simulink model "SingleVehicle_01"  (Simulink 8.8)
settings: Solver=VariableStepAuto  StartTime=0.0  StopTime=35  RelTol=1e-3
undefined symbols (not defined in the file or in its folder): ConnectedBus, DiscIntNeverNeededParam, FromPrescan, IdealSensors, psi, x, y
undefined symbols (not defined in the file): vd
libraries: robotlib x3, PreScanUsefulBlocks x1, PreScanSimulinkLibrary x1
settings Model: LogicAnalyzerSignalOrdering=f5e0fbd6-48e8-44a6-8d7f-3c8f77bb7866  Creator=sgopalswamy  LastModifiedBy=sgopalswamy
settings SolverCC: AutoInsertRateTranBlk=on
settings DataIOCC: LimitDataPoints=off  SaveFormat=Dataset  SignalLoggingSaveFormat=Dataset
settings OptimizationCC: LifeSpan=auto
settings DebuggingCC: MultiTaskRateTransMsg=warning  FcnCallInpInsideContextMsg=error  StateNameClashWarn=none  SFUnexpectedBacktrackingDiag=error  SFNoUnconditionalDefaultTransitionDiag=error  SFExecutionAtInitializationDiag=warning
settings HardwareCC: ProdBitPerPointer=64  ProdBitPerSizeT=64  ProdBitPerPtrDiffT=64  ProdLargestAtomicFloat=Float  ProdIntDivRoundTo=Zero  ProdEndianess=LittleEndian  ProdWordSize=64  ProdHWDeviceType=Intel->x86-64 (Windows64)
settings ModelReferenceCC: PropagateSignalLabelsOutOfModel=on
settings GRTTargetCC: TargetLangStandard=C99 (ISO)  GeneratePreprocessorConditionals=Use local settings  CombineOutputUpdateFcns=on  GRTInterface=off
settings ConfigComp: CovMetricSettings=dwe  CovHtmlReporting=off  CovSaveCumulativeToWorkspaceVar=off  CovSaveSingleToWorkspaceVar=off  CovExternalEMLEnable=on

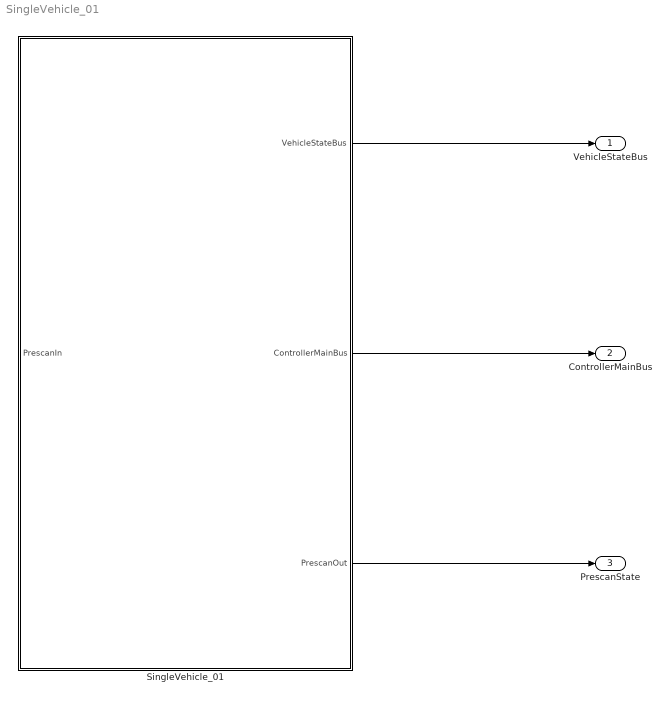
== system SingleVehicle_01 ==
  SingleVehicle_01 : Subsystem  mask{veh_struct=vd}
      mask prompts: veh_struct "Vehicle Parameter Structure"
      mask init:
      | set_param([gcb,'/Monitor/VehicleStateBusStorage'],'VariableName',[get_param(gcb,'MaskValueString'),'_DataVehicleBus']);
      | set_param([gcb,'/Monitor/ControllerMainBusStorage/ArbitratedActuationReqStorage'],'VariableName', ...
      |     [get_param(gcb,'MaskValueString'),'_DataControllerMain_ArbitrationActuationReq']);
      | set_param([gcb,'/Monitor/ControllerMainBusStorage/wpFollowerStorage'],'VariableName', ...
      |     [get_param(gcb,'MaskValueString'),'_DataControllerMain_wpFollower']);
      | set_param([gcb,'/Monitor/ControllerMainBusStorage/finalWayPointStorarge'],'VariableName', ...
      |     [get_param(gcb,'MaskValueString'),'_DataControllerMain_finalWayPoint']);
      | set_param([gcb,'/Monitor/ControllerMainBusStorage/currentWayPointStorage'],'VariableName', ...
      |     [get_param(gcb,'MaskValueString'),'_DataControllerMain_currentWayPoint']);
      | set_param([gcb,'/Monitor/ControllerMainBusStorage/wayPointArrayStorage'],'VariableName', ...
      |     [get_param(gcb,'MaskValueString'),'_DataControllerMain_wayPointArray']);
      | set_param([gcb,'/Monitor/ControllerMainBusStorage/selfAwareessBusStorage'],'VariableName', ...
      |     [get_param(gcb,'MaskValueString'),'_DataControllerMain_selfAwareessBus']);
      | set_param([gcb,'/Monitor/ControllerMainBusStorage/IdealSensorsStorage'],'VariableName', ...
      |     [get_param(gcb,'MaskValueString'),'_DataControllerMain_IdealSensors']);
      | set_param([gcb,'/Monitor/ControllerMainBusStorage/FromPrescanStorage'],'VariableName', ...
      |     [get_param(gcb,'MaskValueString'),'_DataControllerMain_FromPrescan']);
  VehicleStateBus : Outport
  ControllerMainBus : Outport  Port=2
  PrescanState : Outport  Port=3
  wires:
  SingleVehicle_01/1(VehicleStateBus) -> VehicleStateBus/1
  SingleVehicle_01/2(ControllerMainBus) -> ControllerMainBus/1
  SingleVehicle_01/3(PrescanOut) -> PrescanState/1

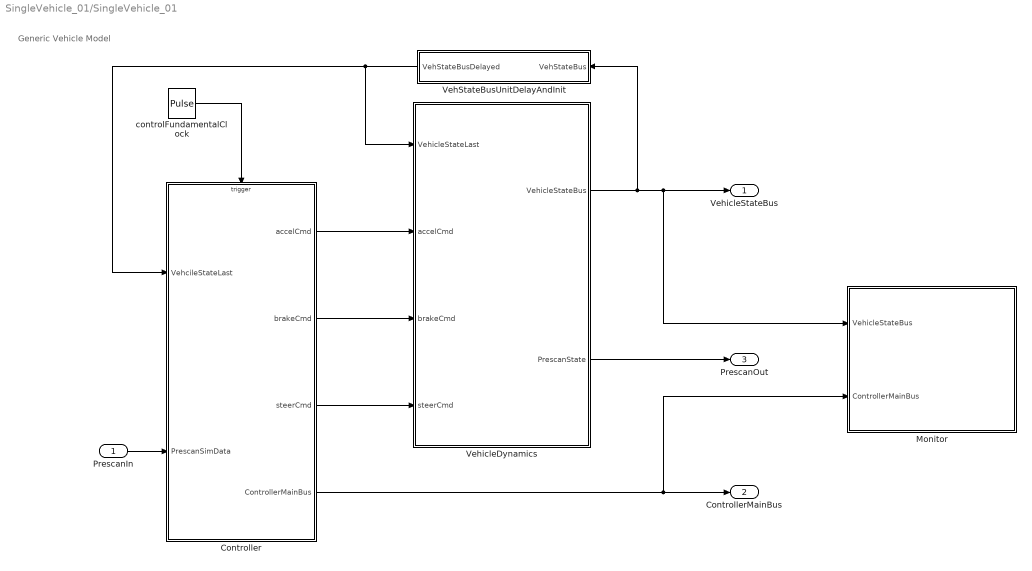
== system SingleVehicle_01/SingleVehicle_01 ==
  note: Generic Vehicle Model
  PrescanIn : Inport
  Controller : Subsystem
  Monitor : Subsystem
  VehStateBusUnitDelayAndInit : Subsystem
  VehicleDynamics : Subsystem
  controlFundamentalClock : DiscretePulseGenerator  PulseType=Time based  Period=veh_struct.CONTROL_OS_SAMPLETIME  PulseWidth=5
  VehicleStateBus : Outport
  ControllerMainBus : Outport  Port=2
  PrescanOut : Outport  Port=3
  wires:
  PrescanIn/1 -> Controller/2(PrescanSimData)
  Controller/1(accelCmd) -> VehicleDynamics/2(accelCmd)
  Controller/2(brakeCmd) -> VehicleDynamics/3(brakeCmd)
  Controller/3(steerCmd) -> VehicleDynamics/4(steerCmd)
  Controller/4(ControllerMainBus) -> Monitor/2(ControllerMainBus), ControllerMainBus/1
  VehicleDynamics/2(PrescanState) -> PrescanOut/1
  VehicleDynamics/1(VehicleStateBus) -> VehStateBusUnitDelayAndInit/1(VehStateBus), VehicleStateBus/1, Monitor/1(VehicleStateBus)
  VehStateBusUnitDelayAndInit/1(VehStateBusDelayed) -> Controller/1(VehcileStateLast), VehicleDynamics/1(VehicleStateLast)
  controlFundamentalClock/1 -> Controller/Trigger

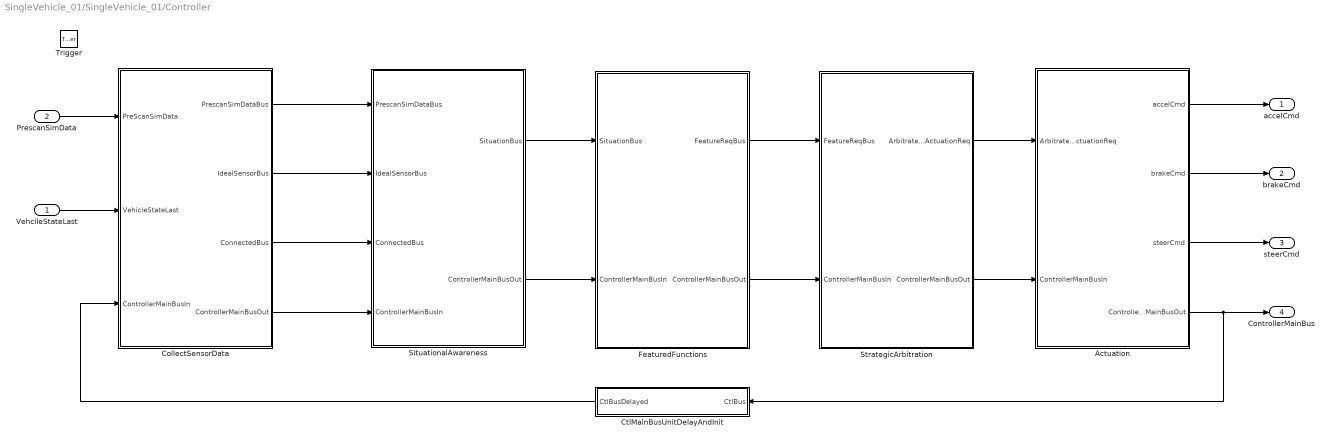
== system SingleVehicle_01/SingleVehicle_01/Controller ==
  VehcileStateLast : Inport
  PrescanSimData : Inport  Port=2
  Trigger : TriggerPort  VariantControl=Variant  PortDimensions=1
  Actuation : Subsystem
  CollectSensorData : Subsystem
  CtlMainBusUnitDelayAndInit : Subsystem
  FeaturedFunctions : Subsystem
  SituationalAwareness : Subsystem
  StrategicArbitration : Subsystem
  accelCmd : Outport
  brakeCmd : Outport  Port=2
  steerCmd : Outport  Port=3
  ControllerMainBus : Outport  Port=4
  wires:
  PrescanSimData/1 -> CollectSensorData/1(PreScanSimData)
  Actuation/1(accelCmd) -> accelCmd/1
  Actuation/2(brakeCmd) -> brakeCmd/1
  Actuation/3(steerCmd) -> steerCmd/1
  StrategicArbitration/1(ArbitratedActuationReq) -> Actuation/1(ArbitratedActuationReq)
  StrategicArbitration/2(ControllerMainBusOut) -> Actuation/2(ControllerMainBusIn)
  FeaturedFunctions/2(ControllerMainBusOut) -> StrategicArbitration/2(ControllerMainBusIn)
  FeaturedFunctions/1(FeatureReqBus) -> StrategicArbitration/1(FeatureReqBus)
  SituationalAwareness/1(SituationBus) -> FeaturedFunctions/1(SituationBus)
  SituationalAwareness/2(ControllerMainBusOut) -> FeaturedFunctions/2(ControllerMainBusIn)
  CollectSensorData/4(ControllerMainBusOut) -> SituationalAwareness/4(ControllerMainBusIn)
  VehcileStateLast/1 -> CollectSensorData/2(VehicleStateLast)
  Actuation/4(ControllerMainBusOut) -> CtlMainBusUnitDelayAndInit/1(CtlBus), ControllerMainBus/1
  CtlMainBusUnitDelayAndInit/1(CtlBusDelayed) -> CollectSensorData/3(ControllerMainBusIn)
  CollectSensorData/1(PrescanSimDataBus) -> SituationalAwareness/1(PrescanSimDataBus)
  CollectSensorData/2(IdealSensorBus) -> SituationalAwareness/2(IdealSensorBus)
  CollectSensorData/3(ConnectedBus) -> SituationalAwareness/3(ConnectedBus)

== system SingleVehicle_01/SingleVehicle_01/Monitor ==
  VehicleStateBus : Inport
  ControllerMainBus : Inport  Port=2
  ControllerMainBusStorage : Subsystem
  VehicleStateBusStorage : ToWorkspace  VariableName=vd_DataVehicleBus  SaveFormat=Timeseries  SampleTime=-1
  wires:
  VehicleStateBus/1 -> VehicleStateBusStorage/1
  ControllerMainBus/1 -> ControllerMainBusStorage/1(ControllerMainBus)

== system SingleVehicle_01/SingleVehicle_01/VehStateBusUnitDelayAndInit ==
  VehStateBus : Inport
  MATLAB Function : MATLAB Function  TreatAsAtomicUnit=on
  Memory : Memory  InheritSampleTime=on
  VehStateBusDelayed : Outport
  wires:
  Memory/1 -> MATLAB Function/1(u)
  VehStateBus/1 -> Memory/1
  MATLAB Function/1(y) -> VehStateBusDelayed/1

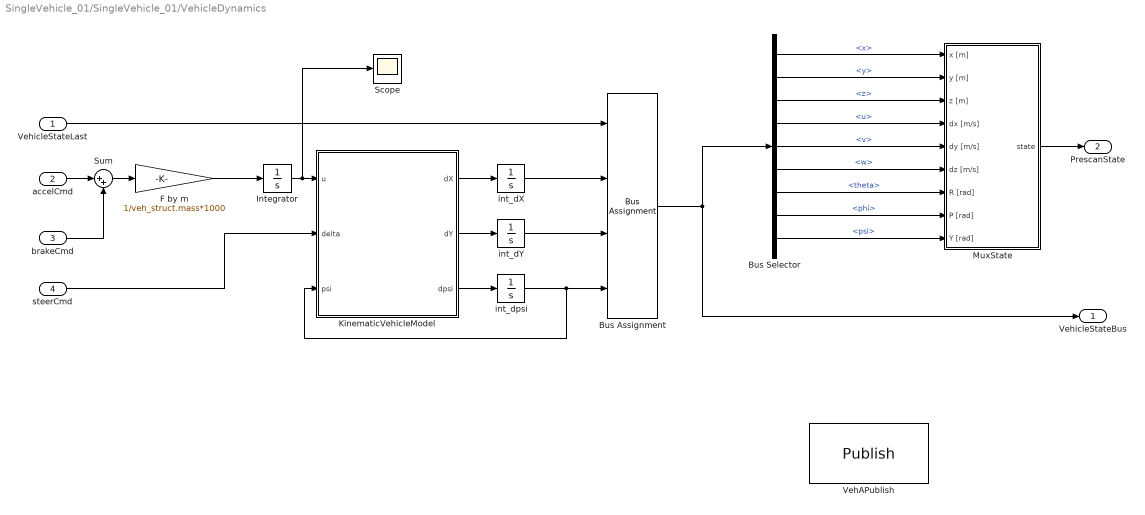
== system SingleVehicle_01/SingleVehicle_01/VehicleDynamics ==
  VehicleStateLast : Inport
  accelCmd : Inport  Port=2
  brakeCmd : Inport  Port=3
  steerCmd : Inport  Port=4
  Bus Assignment : BusAssignment  AssignedSignals=x,y,psi
  Bus Selector : BusSelector  OutputSignals=x,y,z,u,v,w,theta,phi,psi
  F by m : Gain  Gain=1/veh_struct.mass*1000
  Integrator : Integrator  InitialCondition=veh_struct.init.u
  KinematicVehicleModel : MATLAB Function  TreatAsAtomicUnit=on
  MuxState : Subsystem  Tag=MuxState  mask(Empty Dynamics State Block){positioningmode=on, TimeStep=1/20}
      mask prompts: positioningmode "Positioning Mode"; TimeStep "Auto Assigned: Time Step [s]"
      mask help:
      | Build the state of an actor based on user input.
      | The user can either use positioning mode or dynamics mode.
      | - When using positioning mode the position and orientation of the actor are set directly based on the input. Expected input is relative to the initial position and orientation of the actor. It's also possible to specify the velocity of the actor, though this input isn't used, only passed on.
      | - When using dynamics mode the position input is ignored. Expected input is velocity and orientation. The velocity is relative the current orientation of the actor, while orientation is relative to its initial orientation. The position of the actor is calculated based on the velocity and orientation given.
      settings: DeleteFcn=PreScanBlockDeleteFcn;
  Scope : Scope
  Sum : Sum  Inputs=|++
  VehAPublish : robotlib/Publish  SourceLibraryInfo=This block requires Robotics System Toolbox  topicSource=Select from ROS network  topic=/my_topic  messageType=geometry_msgs/Point  messageQueueLength=1
  int_dX : Integrator  InitialCondition=veh_struct.init.X
  int_dY : Integrator  InitialCondition=veh_struct.init.Y
  int_dpsi : Integrator  InitialCondition=veh_struct.init.psi
  VehicleStateBus : Outport
  PrescanState : Outport  Port=2
  wires:
  MuxState/1(state) -> PrescanState/1
  Bus Assignment/1 -> Bus Selector/1, VehicleStateBus/1
  Bus Selector/3 -> MuxState/3(z [m])  "<z>"
  Bus Selector/4 -> MuxState/4(dx [m/s])  "<u>"
  Bus Selector/5 -> MuxState/5(dy [m/s])  "<v>"
  Bus Selector/6 -> MuxState/6(dz [m/s])  "<w>"
  Bus Selector/1 -> MuxState/1(x [m])  "<x>"
  Bus Selector/2 -> MuxState/2(y [m])  "<y>"
  Bus Selector/7 -> MuxState/7(R [rad])  "<theta>"
  Bus Selector/9 -> MuxState/9(Y [rad])  "<psi>"
  Bus Selector/8 -> MuxState/8(P [rad])  "<phi>"
  VehicleStateLast/1 -> Bus Assignment/1
  steerCmd/1 -> KinematicVehicleModel/2(delta)
  accelCmd/1 -> Sum/1
  brakeCmd/1 -> Sum/2
  Sum/1 -> F by m/1
  F by m/1 -> Integrator/1
  Integrator/1 -> Scope/1, KinematicVehicleModel/1(u)
  KinematicVehicleModel/2(dY) -> int_dY/1
  KinematicVehicleModel/1(dX) -> int_dX/1
  KinematicVehicleModel/3(dpsi) -> int_dpsi/1
  int_dX/1 -> Bus Assignment/2
  int_dY/1 -> Bus Assignment/3
  int_dpsi/1 -> Bus Assignment/4, KinematicVehicleModel/3(psi)

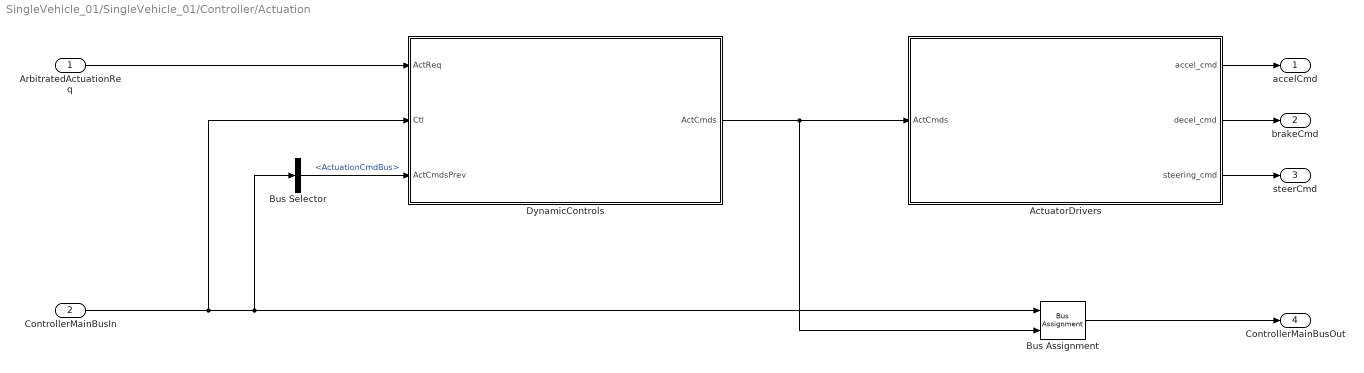
== system SingleVehicle_01/SingleVehicle_01/Controller/Actuation ==
  ArbitratedActuationReq : Inport
  ControllerMainBusIn : Inport  Port=2
  ActuatorDrivers : MATLAB Function  TreatAsAtomicUnit=on
  Bus Assignment : BusAssignment  AssignedSignals=ActuationCmdBus
  Bus Selector : BusSelector  OutputSignals=ActuationCmdBus
  DynamicControls : MATLAB Function  TreatAsAtomicUnit=on
  accelCmd : Outport
  brakeCmd : Outport  Port=2
  steerCmd : Outport  Port=3
  ControllerMainBusOut : Outport  Port=4
  wires:
  ControllerMainBusIn/1 -> DynamicControls/2(Ctl), Bus Assignment/1, Bus Selector/1
  ArbitratedActuationReq/1 -> DynamicControls/1(ActReq)
  Bus Selector/1 -> DynamicControls/3(ActCmdsPrev)  "<ActuationCmdBus>"
  DynamicControls/1(ActCmds) -> ActuatorDrivers/1(ActCmds), Bus Assignment/2
  Bus Assignment/1 -> ControllerMainBusOut/1
  ActuatorDrivers/2(decel_cmd) -> brakeCmd/1
  ActuatorDrivers/1(accel_cmd) -> accelCmd/1
  ActuatorDrivers/3(steering_cmd) -> steerCmd/1

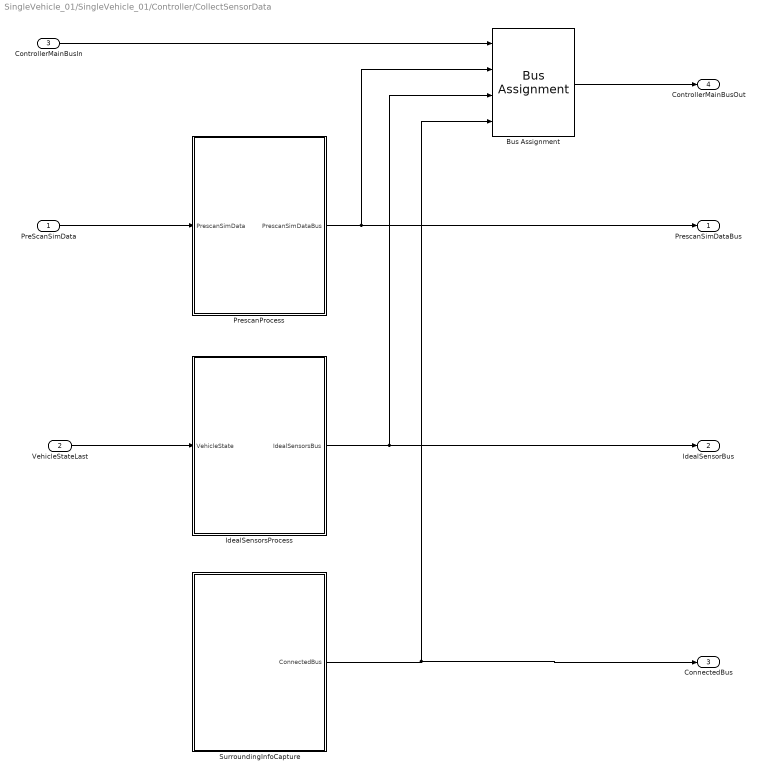
== system SingleVehicle_01/SingleVehicle_01/Controller/CollectSensorData ==
  PreScanSimData : Inport
  VehicleStateLast : Inport  Port=2
  ControllerMainBusIn : Inport  Port=3
  Bus Assignment : BusAssignment  AssignedSignals=FromPrescan,IdealSensors,ConnectedBus
  IdealSensorsProcess : Subsystem
  PrescanProcess : Subsystem
  SurroundingInfoCapture : Subsystem
  PrescanSimDataBus : Outport
  IdealSensorBus : Outport  Port=2
  ConnectedBus : Outport  Port=3
  ControllerMainBusOut : Outport  Port=4
  wires:
  PreScanSimData/1 -> PrescanProcess/1(PrescanSimData)
  PrescanProcess/1(PrescanSimDataBus) -> Bus Assignment/2, PrescanSimDataBus/1
  VehicleStateLast/1 -> IdealSensorsProcess/1(VehicleState)
  IdealSensorsProcess/1(IdealSensorsBus) -> IdealSensorBus/1, Bus Assignment/3
  Bus Assignment/1 -> ControllerMainBusOut/1
  ControllerMainBusIn/1 -> Bus Assignment/1
  SurroundingInfoCapture/1(ConnectedBus) -> ConnectedBus/1, Bus Assignment/4

== system SingleVehicle_01/SingleVehicle_01/Controller/CtlMainBusUnitDelayAndInit ==
  CtlBus : Inport
  MATLAB Function : MATLAB Function  TreatAsAtomicUnit=on
  Memory : Memory  InheritSampleTime=on
  CtlBusDelayed : Outport
  wires:
  Memory/1 -> MATLAB Function/1(u)
  CtlBus/1 -> Memory/1
  MATLAB Function/1(y) -> CtlBusDelayed/1

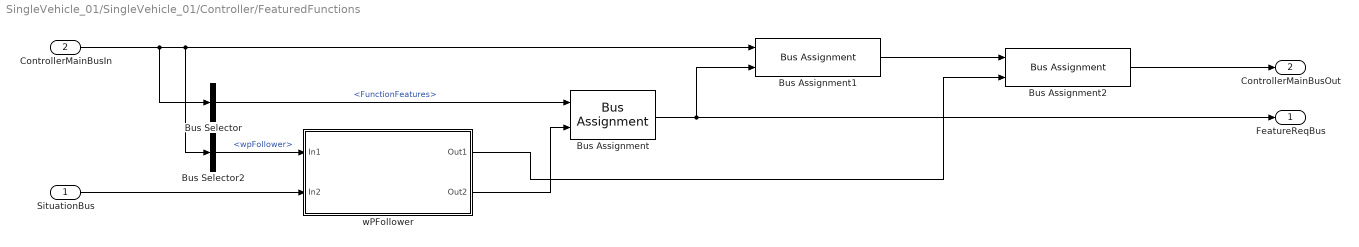
== system SingleVehicle_01/SingleVehicle_01/Controller/FeaturedFunctions ==
  SituationBus : Inport
  ControllerMainBusIn : Inport  Port=2
  Bus Assignment : BusAssignment  AssignedSignals=wpFollower
  Bus Assignment1 : BusAssignment  AssignedSignals=FunctionFeatures
  Bus Assignment2 : BusAssignment  AssignedSignals=situationBus
  Bus Selector : BusSelector  OutputSignals=FunctionFeatures
  Bus Selector2 : BusSelector  OutputSignals=FunctionFeatures.wpFollower
  wPFollower : Subsystem
  FeatureReqBus : Outport
  ControllerMainBusOut : Outport  Port=2
  wires:
  ControllerMainBusIn/1 -> Bus Selector/1, Bus Selector2/1, Bus Assignment1/1
  Bus Selector/1 -> Bus Assignment/1  "<FunctionFeatures>"
  Bus Assignment/1 -> Bus Assignment1/2, FeatureReqBus/1
  Bus Assignment1/1 -> Bus Assignment2/1
  Bus Assignment2/1 -> ControllerMainBusOut/1
  Bus Selector2/1 -> wPFollower/1(In1)  "<wpFollower>"
  SituationBus/1 -> wPFollower/2(In2)
  wPFollower/1(Out1) -> Bus Assignment2/2
  wPFollower/2(Out2) -> Bus Assignment/2

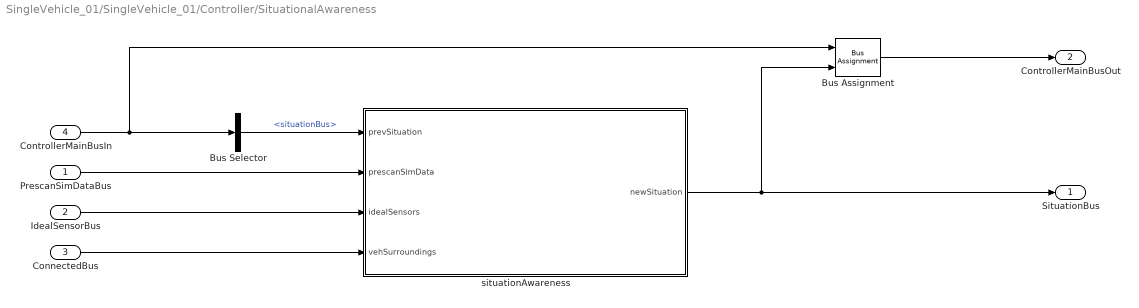
== system SingleVehicle_01/SingleVehicle_01/Controller/SituationalAwareness ==
  PrescanSimDataBus : Inport
  IdealSensorBus : Inport  Port=2
  ConnectedBus : Inport  Port=3
  ControllerMainBusIn : Inport  Port=4
  Bus Assignment : BusAssignment  AssignedSignals=situationBus
  Bus Selector : BusSelector  OutputSignals=situationBus
  situationAwareness : MATLAB Function  TreatAsAtomicUnit=on
  SituationBus : Outport
  ControllerMainBusOut : Outport  Port=2
  wires:
  ControllerMainBusIn/1 -> Bus Assignment/1, Bus Selector/1
  Bus Selector/1 -> situationAwareness/1(prevSituation)  "<situationBus>"
  PrescanSimDataBus/1 -> situationAwareness/2(prescanSimData)
  IdealSensorBus/1 -> situationAwareness/3(idealSensors)
  situationAwareness/1(newSituation) -> Bus Assignment/2, SituationBus/1
  Bus Assignment/1 -> ControllerMainBusOut/1
  ConnectedBus/1 -> situationAwareness/4(vehSurroundings)

== system SingleVehicle_01/SingleVehicle_01/Controller/StrategicArbitration ==
  FeatureReqBus : Inport
  ControllerMainBusIn : Inport  Port=2
  Arbitration : MATLAB Function  TreatAsAtomicUnit=on
  Bus Assignment : BusAssignment  AssignedSignals=ArbitratedActuationReq
  ArbitratedActuationReq : Outport
  ControllerMainBusOut : Outport  Port=2
  wires:
  ControllerMainBusIn/1 -> Bus Assignment/1
  FeatureReqBus/1 -> Arbitration/1(FunctionFeatures)
  Arbitration/1(ArbitratedReq) -> Bus Assignment/2, ArbitratedActuationReq/1
  Bus Assignment/1 -> ControllerMainBusOut/1

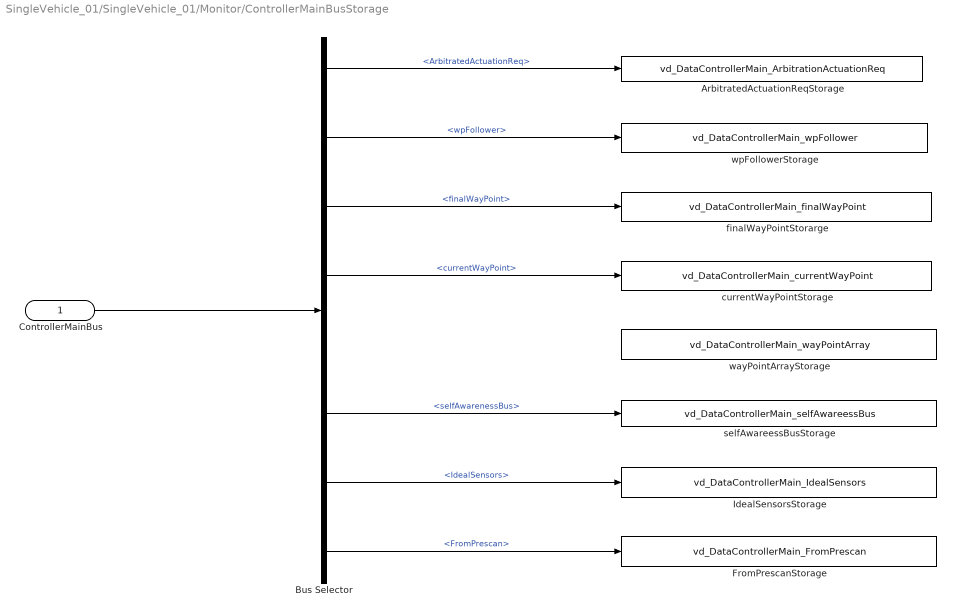
== system SingleVehicle_01/SingleVehicle_01/Monitor/ControllerMainBusStorage ==
  ControllerMainBus : Inport
  ArbitratedActuationReqStorage : ToWorkspace  VariableName=vd_DataControllerMain_ArbitrationActuationReq  SaveFormat=Timeseries  SampleTime=-1
  Bus Selector : BusSelector  OutputSignals=ArbitratedActuationReq,FunctionFeatures.wpFollower,situationBus.wP.finalWayPoint,situationBus.wP.currentWayPoint,situationBus.wP.wayPointArray,situationBus.selfAwarenessBus,IdealSensors,FromPrescan
  FromPrescanStorage : ToWorkspace  VariableName=vd_DataControllerMain_FromPrescan  SaveFormat=Timeseries  SampleTime=-1
  IdealSensorsStorage : ToWorkspace  VariableName=vd_DataControllerMain_IdealSensors  SaveFormat=Timeseries  SampleTime=-1
  currentWayPointStorage : ToWorkspace  VariableName=vd_DataControllerMain_currentWayPoint  SaveFormat=Timeseries  SampleTime=-1
  finalWayPointStorarge : ToWorkspace  VariableName=vd_DataControllerMain_finalWayPoint  SaveFormat=Timeseries  SampleTime=-1
  selfAwareessBusStorage : ToWorkspace  VariableName=vd_DataControllerMain_selfAwareessBus  SaveFormat=Timeseries  SampleTime=-1
  wayPointArrayStorage : ToWorkspace  VariableName=vd_DataControllerMain_wayPointArray  SampleTime=-1
  wpFollowerStorage : ToWorkspace  VariableName=vd_DataControllerMain_wpFollower  SaveFormat=Timeseries  SampleTime=-1
  wires:
  ControllerMainBus/1 -> Bus Selector/1
  Bus Selector/1 -> ArbitratedActuationReqStorage/1  "<ArbitratedActuationReq>"
  Bus Selector/2 -> wpFollowerStorage/1  "<wpFollower>"
  Bus Selector/3 -> finalWayPointStorarge/1  "<finalWayPoint>"
  Bus Selector/8 -> FromPrescanStorage/1  "<FromPrescan>"
  Bus Selector/6 -> selfAwareessBusStorage/1  "<selfAwarenessBus>"
  Bus Selector/4 -> currentWayPointStorage/1  "<currentWayPoint>"
  Bus Selector/7 -> IdealSensorsStorage/1  "<IdealSensors>"

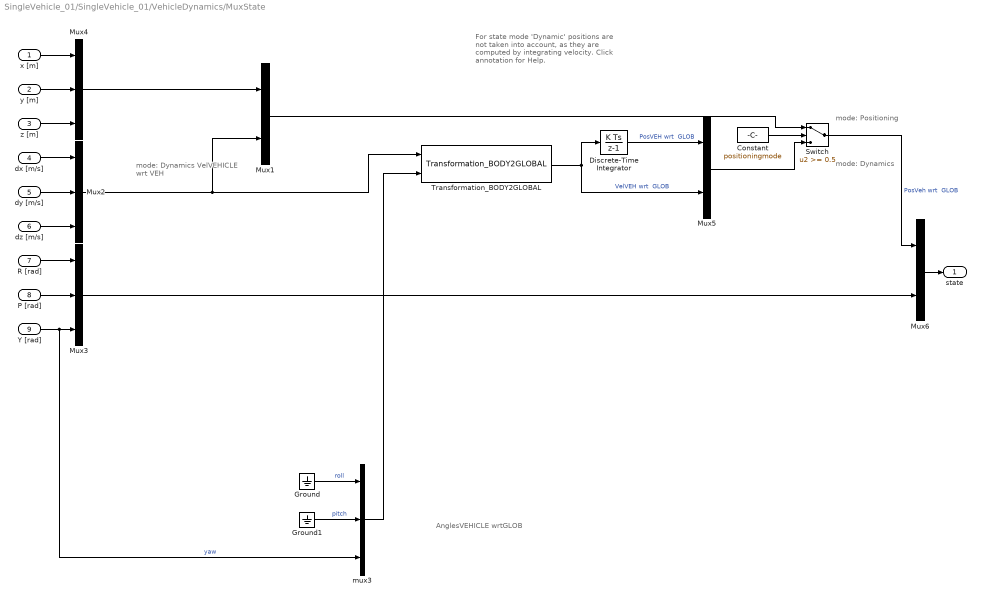
== system SingleVehicle_01/SingleVehicle_01/VehicleDynamics/MuxState ==
  note: mode: Dynamics
  note: mode: Positioning
  note: mode: Dynamics
      | VelVEHICLE
      | wrt VEH
  note: AnglesVEHICLE
      | wrtGLOB
  note: For state mode 'Dynamic' positions
      | are not taken into account, as they
      | are computed by integrating velocity.
      | Click annotation for Help.
  x [m] : Inport  SampleTime=TimeStep
  y [m] : Inport  Port=2  SampleTime=TimeStep
  z [m] : Inport  Port=3  SampleTime=TimeStep
  dx [m/s] : Inport  Port=4  SampleTime=TimeStep
  dy [m/s] : Inport  Port=5  SampleTime=TimeStep
  dz [m/s] : Inport  Port=6  SampleTime=TimeStep
  R [rad] : Inport  Port=7  SampleTime=TimeStep
  P [rad] : Inport  Port=8  SampleTime=TimeStep
  Y [rad] : Inport  Port=9  SampleTime=TimeStep
  Constant : Constant  DisableCoverage=on  Value=positioningmode
  Discrete-Time Integrator : DiscreteIntegrator  SampleTime=TimeStep  ICPrevOutput=DiscIntNeverNeededParam  ICPrevScaledInput=DiscIntNeverNeededParam
  Ground : Ground
  Ground1 : Ground
  Mux1 : Mux  Inputs=[3 3]
  Mux2 : Mux  Inputs=3
  Mux3 : Mux  Inputs=3
  Mux4 : Mux  Inputs=3
  Mux5 : Mux  Inputs=[3 3]
  Mux6 : Mux  Inputs=[6 3]
  Switch : Switch  Threshold=0.5
  Transformation_BODY2GLOBAL : PreScanSimulinkLibrary/Simple_Vehicle_Dynamics/Chassis/MuxDynState/Transformation_BODY2GLOBAL
  mux3 : Mux  Inputs=3
  state : Outport
  wires:
  Constant/1 -> Switch/2
  Mux6/1 -> state/1
  Mux4/1 -> Mux1/1
  Mux5/1 -> Switch/3
  Mux1/1 -> Switch/1
  Switch/1 -> Mux6/1  "PosVeh wrt  GLOB"
  P [rad]/1 -> Mux3/2
  R [rad]/1 -> Mux3/1
  dz [m/s]/1 -> Mux2/3
  dy [m/s]/1 -> Mux2/2
  dx [m/s]/1 -> Mux2/1
  z [m]/1 -> Mux4/3
  y [m]/1 -> Mux4/2
  x [m]/1 -> Mux4/1
  Ground1/1 -> mux3/2  "pitch"
  Y [rad]/1 -> mux3/3, Mux3/3  "yaw"
  Mux3/1 -> Mux6/2
  Transformation_BODY2GLOBAL/1 -> Discrete-Time Integrator/1, Mux5/2  "VelVEH wrt  GLOB"
  mux3/1 -> Transformation_BODY2GLOBAL/2
  Ground/1 -> mux3/1  "roll"
  Mux2/1 -> Mux1/2, Transformation_BODY2GLOBAL/1
  Discrete-Time Integrator/1 -> Mux5/1  "PosVEH wrt  GLOB"

== system SingleVehicle_01/SingleVehicle_01/Controller/CollectSensorData/IdealSensorsProcess ==
  VehicleState : Inport
  Bus Creator : BusCreator  Inputs=12  OutDataTypeStr=Bus: VehState
  Bus Selector : BusSelector  OutputSignals=x,y,z,theta,phi,psi,u,v,w,dtheta,dphi,dpsi
  IdealSensorsBus : Outport
  wires:
  VehicleState/1 -> Bus Selector/1
  Bus Selector/1 -> Bus Creator/1  "<x>"
  Bus Selector/8 -> Bus Creator/8  "<v>"
  Bus Selector/7 -> Bus Creator/7  "<u>"
  Bus Selector/10 -> Bus Creator/10  "<dtheta>"
  Bus Selector/11 -> Bus Creator/11  "<dphi>"
  Bus Selector/6 -> Bus Creator/6  "<psi>"
  Bus Selector/4 -> Bus Creator/4  "<theta>"
  Bus Selector/9 -> Bus Creator/9  "<w>"
  Bus Selector/2 -> Bus Creator/2  "<y>"
  Bus Selector/5 -> Bus Creator/5  "<phi>"
  Bus Selector/12 -> Bus Creator/12  "<dpsi>"
  Bus Selector/3 -> Bus Creator/3  "<z>"
  Bus Creator/1 -> IdealSensorsBus/1

== system SingleVehicle_01/SingleVehicle_01/Controller/CollectSensorData/PrescanProcess ==
  PrescanSimData : Inport
  Bus Creator : BusCreator  Inputs=12  OutDataTypeStr=Bus: PrescanSimData
      settings: InheritFromInputs=off
  SELF_Demux : Subsystem  Tag=DemuxSELF  mask(PreScan Demux Block:){}
      settings: DeleteFcn=PreScanBlockDeleteFcn;
      mask Display:
      | port_label('output',1,'x [m]')
      | port_label('output',2,'y [m]')
      | port_label('output',3,'z [m]','texmode','on')
      | port_label('output',4,'Rotx [deg]','texmode','on')
      | port_label('output',5,'Roty [deg]','texmode','on')
      | port_label('output',6,'Rotz [deg]','texmode','on')
      | port_label('output',7,'GPS lat [deg]','texmode','on')
      | port_label('output',8,'GPS long [deg]','texmode','on')
      | port_label('output',9,'GPS alt [m]','texmode','on')
      | port_label('output',10,'Velocity [m/s]')
      | port_label('output',11,'Heading [deg]')
      | port_label('output',12,'Yaw rate [deg/s]')
  PrescanSimDataBus : Outport
  wires:
  SELF_Demux/1(x [m]) -> Bus Creator/1  "x"
  PrescanSimData/1 -> SELF_Demux/1(SELF)
  Bus Creator/1 -> PrescanSimDataBus/1
  SELF_Demux/2(y [m]) -> Bus Creator/2  "y"
  SELF_Demux/3(z [m]) -> Bus Creator/3  "z"
  SELF_Demux/4(rotx [deg]) -> Bus Creator/4  "Rotx"
  SELF_Demux/5(roty [deg]) -> Bus Creator/5  "Roty"
  SELF_Demux/9(GPS alt [m]) -> Bus Creator/9  "GPS_alt"
  SELF_Demux/8(GPS long [deg]) -> Bus Creator/8  "GPS_long"
  SELF_Demux/10(velocity [m/s]) -> Bus Creator/10  "u"
  SELF_Demux/6(rotz [deg]) -> Bus Creator/6  "Rotz"
  SELF_Demux/7(GPS lat [deg]) -> Bus Creator/7  "GPS_lat"
  SELF_Demux/11(heading [deg]) -> Bus Creator/11  "heading"
  SELF_Demux/12(yaw rate [deg/s]) -> Bus Creator/12  "Yaw_rate"

== system SingleVehicle_01/SingleVehicle_01/Controller/CollectSensorData/SurroundingInfoCapture ==
  Bus Creator : BusCreator  Inputs=2  OutDataTypeStr=Bus: ConnectedBus
  Bus Creator1 : BusCreator  Inputs=3  OutDataTypeStr=Bus: ObjectBus
  Bus Selector1 : BusSelector  OutputSignals=X,Y,Z
  NumberObject : Constant  Value=2
  Terminator : Terminator
  VehicleB_FromSim_Object2 : robotlib/Subscribe  SourceLibraryInfo=This block requires Robotics System Toolbox  topicSource=Select from ROS network  topic=/my_topic  messageType=geometry_msgs/Point  sampleTime=-1  messageQueueLength=1
  VehicleC_RCVehicle_Object1 : robotlib/Subscribe  SourceLibraryInfo=This block requires Robotics System Toolbox  topicSource=Select from ROS network  topic=/my_topic  messageType=geometry_msgs/Point  sampleTime=-1  messageQueueLength=1
  ConnectedBus : Outport
  wires:
  Bus Creator/1 -> ConnectedBus/1
  VehicleC_RCVehicle_Object1/2 -> Bus Selector1/1
  Bus Selector1/1 -> Bus Creator1/1  "<X>"
  Bus Selector1/2 -> Bus Creator1/2  "<Y>"
  Bus Selector1/3 -> Bus Creator1/3  "<Z>"
  NumberObject/1 -> Bus Creator/2  "NumberObjects"
  VehicleC_RCVehicle_Object1/1 -> Terminator/1
  Bus Creator1/1 -> Bus Creator/1  "ObjectBus"

== system SingleVehicle_01/SingleVehicle_01/Controller/FeaturedFunctions/wPFollower ==
  In1 : Inport
  In2 : Inport  Port=2
  calcDesdCmds : MATLAB Function  TreatAsAtomicUnit=on
  defineWayPointsNewWay : MATLAB Function  TreatAsAtomicUnit=on
  defineWayPointsOldWay : MATLAB Function  TreatAsAtomicUnit=on
  Out1 : Outport
  Out2 : Outport  Port=2
  wires:
  In2/1 -> defineWayPointsOldWay/2(prevSituation)
  In1/1 -> defineWayPointsOldWay/1(prevWpAction)
  defineWayPointsOldWay/1(wpAction) -> Out2/1
  defineWayPointsOldWay/2(newSituation) -> Out1/1

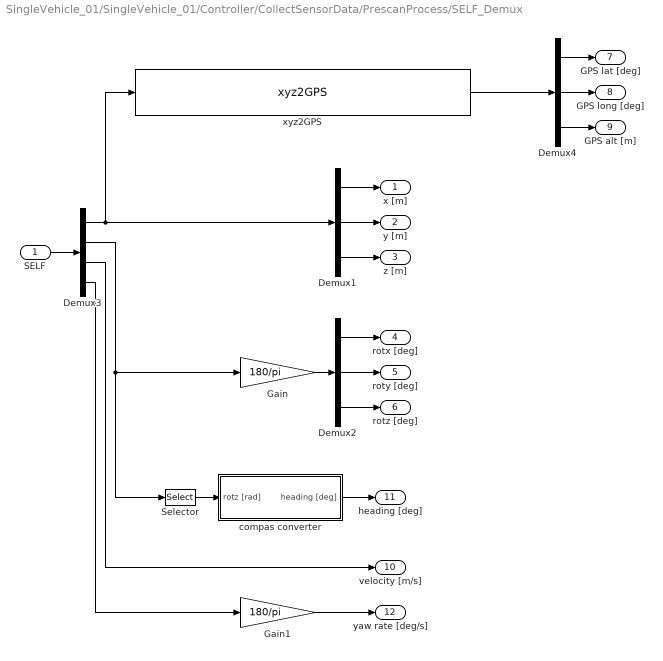
== system SingleVehicle_01/SingleVehicle_01/Controller/CollectSensorData/PrescanProcess/SELF_Demux ==
  SELF : Inport
  Demux1 : Demux  Outputs=3
  Demux2 : Demux  Outputs=3
  Demux3 : Demux  Outputs=[3 3 1 1]
  Demux4 : Demux  Outputs=3
  Gain : Gain  Gain=180/pi
  Gain1 : Gain  Gain=180/pi
  Selector : Selector  InputPortWidth=3  IndexOptions=Index vector (dialog)  Indices=[3]  OutputSizes=1
  compas converter : Subsystem
  xyz2GPS : PreScanUsefulBlocks/xyz2GPS  CoordinateCount=1  GPS_base=[0.000000 0.000000 0.000]
  x [m] : Outport
  y [m] : Outport  Port=2
  z [m] : Outport  Port=3
  rotx [deg] : Outport  Port=4
  roty [deg] : Outport  Port=5
  rotz [deg] : Outport  Port=6
  GPS lat [deg] : Outport  Port=7
  GPS long [deg] : Outport  Port=8
  GPS alt [m] : Outport  Port=9
  velocity [m/s] : Outport  Port=10
  heading [deg] : Outport  Port=11
  yaw rate [deg/s] : Outport  Port=12
  wires:
  Demux3/4 -> Gain1/1
  Gain1/1 -> yaw rate [deg/s]/1
  Demux3/3 -> velocity [m/s]/1
  compas converter/1(heading [deg]) -> heading [deg]/1
  xyz2GPS/1 -> Demux4/1
  Demux4/3 -> GPS alt [m]/1
  Demux4/2 -> GPS long [deg]/1
  Demux4/1 -> GPS lat [deg]/1
  Demux3/2 -> Gain/1, Selector/1
  Demux3/1 -> xyz2GPS/1, Demux1/1
  SELF/1 -> Demux3/1
  Demux2/3 -> rotz [deg]/1
  Demux2/2 -> roty [deg]/1
  Demux2/1 -> rotx [deg]/1
  Demux1/3 -> z [m]/1
  Demux1/2 -> y [m]/1
  Demux1/1 -> x [m]/1
  Gain/1 -> Demux2/1
  Selector/1 -> compas converter/1(rotz [rad])

== system SingleVehicle_01/SingleVehicle_01/Controller/CollectSensorData/PrescanProcess/SELF_Demux/compas converter ==
  rotz [rad] : Inport
  cart2compas : Subsystem
  rad2deg : Gain  Gain=180/pi
  heading [deg] : Outport
  wires:
  cart2compas/1(heading [deg]) -> heading [deg]/1
  rotz [rad]/1 -> rad2deg/1
  rad2deg/1 -> cart2compas/1(Angle [deg])

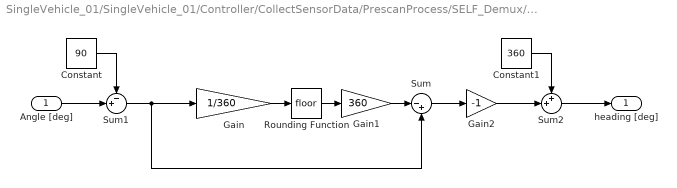
== system SingleVehicle_01/SingleVehicle_01/Controller/CollectSensorData/PrescanProcess/SELF_Demux/compas converter/cart2compas ==
  Angle [deg] : Inport
  Constant : Constant  Value=90
  Constant1 : Constant  Value=360
  Gain : Gain  Gain=1/360
  Gain1 : Gain  Gain=360
  Gain2 : Gain  Gain=-1
  Rounding Function : Rounding
  Sum : Sum  Inputs=|-+
  Sum1 : Sum  Inputs=-+|
  Sum2 : Sum  Inputs=++|
  heading [deg] : Outport
  wires:
  Sum2/1 -> heading [deg]/1
  Constant1/1 -> Sum2/1
  Gain2/1 -> Sum2/2
  Constant/1 -> Sum1/1
  Sum1/1 -> Sum/2, Gain/1
  Sum/1 -> Gain2/1
  Angle [deg]/1 -> Sum1/2
  Gain1/1 -> Sum/1
  Rounding Function/1 -> Gain1/1
  Gain/1 -> Rounding Function/1

== matlab function SingleVehicle_01/Controller/CtlMainBusUnitDelayAndInit/MATLAB Function ==
  data: u input double; y output Bus: ControllerMainBus; veh_struct parameter double
function y = DelayAndInitCtlBus(u, veh_struct)
coder.extrinsic('exist')
persistent a

y0 = struct;

y0.ActuationCmdBus = struct;
y0.ActuationCmdBus.steering_cmd = 0;
y0.ActuationCmdBus.decel_cmd = 0;
y0.ActuationCmdBus.accel_cmd = 0;

y0.ArbitratedActuationReq = struct;
y0.ArbitratedActuationReq.v_des = 0;
y0.ArbitratedActuationReq.a_des = 0;
y0.ArbitratedActuationReq.psi_des = 0;
y0.ArbitratedActuationReq.dpsi_des = 0;


y0.FunctionFeatures = struct;
y0.FunctionFeatures.wpFollower = struct;
y0.FunctionFeatures.wpFollower.v_des = 0;
y0.FunctionFeatures.wpFollower.a_des = 0;
y0.FunctionFeatures.wpFollower.psi_des = 0;
y0.FunctionFeatures.wpFollower.dpsi_des = 0;


y0.situationBus = struct;
y0.situationBus.wP = struct;

y0.situationBus.wP.finalWayPoint = struct;
y0.situationBus.wP.finalWayPoint.x = 0;
y0.situationBus.wP.finalWayPoint.y = 0;
y0.situationBus.wP.finalWayPoint.z = 0;
y0.situationBus.wP.finalWayPoint.treach = 0;

y0.situationBus.wP.currentWayPoint = struct;
y0.situationBus.wP.currentWayPoint.x = 0;
y0.situationBus.wP.currentWayPoint.y = 0;
y0.situationBus.wP.currentWayPoint.z = 0;
y0.situationBus.wP.currentWayPoint.treach = 0;

y0.situationBus.wP.finalWayPointIndex = uint16(1);
y0.situationBus.wP.currentWayPointIndex = uint16(10);

%y0.situationBus.wP.wayPointArray = struct;
wPArray = struct;
wPArray.x = 0;
wPArray.y = 0;
wPArray.z = 0;
wPArray.treach = 0;
y0.situationBus.wP.wayPointArray = repmat(wPArray,100,1);


y0.situationBus.selfAwarenessBus = struct;
y0.situationBus.selfAwarenessBus.x = 0;
y0.situationBus.selfAwarenessBus.y = 0;
y0.situationBus.selfAwarenessBus.z = 0;
y0.situationBus.selfAwarenessBus.theta = 0;
y0.situationBus.selfAwarenessBus.phi = 0;
y0.situationBus.selfAwarenessBus.psi = 0;
y0.situationBus.selfAwarenessBus.u = 0;
y0.situationBus.selfAwarenessBus.v = 0;
y0.situationBus.selfAwarenessBus.w = 0;
y0.situationBus.selfAwarenessBus.dtheta = 0;
y0.situationBus.selfAwarenessBus.dphi = 0;
y0.situationBus.selfAwarenessBus.dpsi = 0;
y0.IdealSensors = struct;
y0.IdealSensors.x = 0;
y0.IdealSensors.y = 0;
y0.IdealSensors.z = 0;
y0.IdealSensors.theta = 0;
y0.IdealSensors.phi = 0;
y0.IdealSensors.psi = 0;
y0.IdealSensors.u = 0;
y0.IdealSensors.v = 0;
y0.IdealSensors.w = 0;
y0.IdealSensors.dtheta = 0;
y0.IdealSensors.dphi = 0;
y0.IdealSensors.dpsi = 0;
y0.FromPrescan = struct;
y0.FromPrescan.x = 0;
y0.FromPrescan.y = 0;
y0.FromPrescan.z = 0;
y0.FromPrescan.Rotx = 0;
y0.FromPrescan.Roty = 0;
y0.FromPrescan.Rotz = 0;
y0.FromPrescan.GPS_lat = 0;
y0.FromPrescan.GPS_long = 0;
y0.FromPrescan.u = 0;
y0.FromPrescan.GPS_alt = 0;
y0.FromPrescan.heading = 0;
y0.FromPrescan.Yaw_rate = 0;

y0.ConnectedBus = struct;
y0.ConnectedBus.ObjectBus = struct;
y0.ConnectedBus.ObjectBus.x = 0;
y0.ConnectedBus.ObjectBus.y = 0;
y0.ConnectedBus.ObjectBus.z = 0;
y0.ConnectedBus.NumberObjects = 0;



if isempty(a)
    a = 1;
    y = y0;
    y.situationBus.wP.wayPointArray = veh_struct.initialWayPointsArray;
    y.situationBus.wP.currentWayPointIndex = veh_struct.initialCurrentWayPointIndex;
    y.situationBus.wP.finalWayPointIndex = veh_struct.initialFinalWayPointIndex;

else
    y = u;
end

== matlab function SingleVehicle_01/VehStateBusUnitDelayAndInit/MATLAB Function ==
  data: u input double; y output Bus: VehState
function y = DelayAndInitVehState(u)
persistent a
y0 = struct;
y0.x = 1;
y0.y = 2;
y0.z = 0;
y0.theta = 0;
y0.phi = 0;
y0.psi = 0;
y0.u = 0;
y0.v = 0;
y0.w = 0;
y0.dtheta = 0;
y0.dphi = 0;
y0.dpsi = 0;

%y0 = VehState_MATLABStruct;
if isempty(a)
    a = 1;
    y = y0;
else
    y = u;
end

== matlab function SingleVehicle_01/Controller/SituationalAwareness/situationAwareness ==
  data: prevSituation input Bus: situationBus; newSituation output Bus: situationBus; prescanSimData input Bus: PrescanSimData; idealSensors input Bus: VehState; veh_struct parameter double; vehSurroundings input double
function newSituation = calcSituationAwareness(prevSituation,prescanSimData,idealSensors, veh_struct, vehSurroundings)

newSituation = prevSituation;


newSituation.selfAwarenessBus.x = idealSensors.x;
newSituation.selfAwarenessBus.y = idealSensors.y;
newSituation.selfAwarenessBus.z = idealSensors.z;
newSituation.selfAwarenessBus.theta = idealSensors.theta;
newSituation.selfAwarenessBus.phi = idealSensors.phi;
newSituation.selfAwarenessBus.psi = idealSensors.psi;
newSituation.selfAwarenessBus.u = idealSensors.u;
newSituation.selfAwarenessBus.v = idealSensors.v;
newSituation.selfAwarenessBus.w = idealSensors.w;
newSituation.selfAwarenessBus.dtheta = idealSensors.dtheta;
newSituation.selfAwarenessBus.dphi = idealSensors.dphi;
newSituation.selfAwarenessBus.dpsi = idealSensors.dpsi;

for i = 1: ContorllerBus.ConnectedBus.NumberObjects
    newSituation.contextualAwareness.ObjectBus(1).x = ControllerBus.ConnectedBus.ObjectBus(1).x;
    newSituation.contextualAwareness.ObjectBus(1).x = ControllerBus.ConnectedBus.ObjectBus(1).y;
    newSituation.contextualAwareness.ObjectBus(1).x = ControllerBus.ConnectedBus.ObjectBus(1).z;
end


end

== matlab function SingleVehicle_01/Controller/FeaturedFunctions/wPFollower/defineWayPointsOldWay ==
  data: prevWpAction input Bus: wpFollower; prevSituation input Bus: situationBus; wpAction output Bus: wpFollower; veh_struct parameter double; newSituation output Bus: situationBus
function [wpAction, newSituation] = wpFollower(prevWpAction, prevSituation, veh_struct)


%waypoint Definition
currentIndex = prevSituation.wP.currentWayPointIndex;
if currentIndex < 1
    currentIndex = uint16(1);
end
finalIndex = prevSituation.wP.finalWayPointIndex;

xd = prevSituation.wP.wayPointArray(currentIndex).x;
yd = prevSituation.wP.wayPointArray(currentIndex).y;
xa = prevSituation.selfAwarenessBus.x;
ya = prevSituation.selfAwarenessBus.y;
howClose = norm([xd-xa, yd-ya]);

if howClose < veh_struct.wpControl.wayPointThreshold
    if (currentIndex == finalIndex)
        currentIndex = uint16(1);
    else
        currentIndex = uint16(currentIndex + 1);
    end
end

newSituation = prevSituation;
newSituation.wP.currentWayPointIndex = uint16(currentIndex);
newSituation.wP.currentWayPoint.x = newSituation.wP.wayPointArray(currentIndex).x;
newSituation.wP.currentWayPoint.y = newSituation.wP.wayPointArray(currentIndex).y;
newSituation.wP.currentWayPoint.z = newSituation.wP.wayPointArray(currentIndex).z;
newSituation.wP.currentWayPoint.treach = newSituation.wP.wayPointArray(currentIndex).treach;


%New Way POint Definition

newSituation = prevSituation;
newSituation.wP.currentWayPointIndex = uint16(currentIndex);
newSituation.wP.currentWayPoint.x = ControllerBus.ConnectedBus.ObjectBus.x;
newSituation.wP.currentWayPoint.y = ControllerBus.ConnectedBus.ObjectBus.y;
newSituation.wP.currentWayPoint.z = ControllerBus.ConnectedBus.ObjectBus.z;
newSituation.wP.currentWayPoint.treach = 0;


%wayPoint Following Algorithm

v_des_raw = min(veh_struct.wpControl.v_des_max, howClose / veh_struct.wpControl.howClose_saturate * veh_struct.wpControl.v_des_max);
psi_des_raw = atan2((yd-ya),(xd-xa));

% if psi_des_raw < 0
%     
%     dbg = 1;
%     
% end
    

v_des_old = prevWpAction.v_des;
psi_des_old = prevWpAction.psi_des;

a_des = veh_struct.wpControl.v_des_filter.lambda * (v_des_raw - v_des_old);
v_des = v_des_old + veh_struct.CONTROL_OS_SAMPLETIME * a_des;

dpsi_des = veh_struct.wpControl.psi_des_filter.lambda * (psi_des_raw - psi_des_old);
psi_des = psi_des_old + veh_struct.CONTROL_OS_SAMPLETIME * dpsi_des;
% psi_des = mod(psi_des, 2 * pi);


wpAction.v_des = v_des;
wpAction.a_des = a_des;
wpAction.psi_des = psi_des;
wpAction.dpsi_des = dpsi_des;

end

== matlab function SingleVehicle_01/Controller/StrategicArbitration/Arbitration ==
  data: FunctionFeatures input Bus: FunctionFeatures; ArbitratedReq output Bus: ArbitratedActuationReq
function ArbitratedReq = Arbitrate(FunctionFeatures)

ArbitratedReq.v_des = FunctionFeatures.wpFollower.v_des;
ArbitratedReq.a_des = FunctionFeatures.wpFollower.a_des;
ArbitratedReq.psi_des = FunctionFeatures.wpFollower.psi_des;
ArbitratedReq.dpsi_des = FunctionFeatures.wpFollower.dpsi_des;

end

== matlab function SingleVehicle_01/Controller/Actuation/DynamicControls ==
  data: ActReq input Bus: ArbitratedActuationReq; Ctl input Bus: ControllerMainBus; ActCmds output Bus: ActuationCmdBus; ActCmdsPrev input Bus: ActuationCmdBus
function ActCmds  = fcn(ActReq, Ctl, ActCmdsPrev)

v_des = ActReq.v_des;
a_des = ActReq.a_des;
psi_des = ActReq.psi_des;
dpsi_des = ActReq.dpsi_des;

% ActCmds = ActCmdsPrev;
% ActCmds.accel_cmd = 0;
% ActCmds.decel_cmd = 0;
% ActCmds.steering_cmd = 0.1;

ActCmds = ActCmdsPrev;

if a_des >= 0
    ActCmds.accel_cmd = ActReq.a_des;
    ActCmds.decel_cmd = 0;
else
    ActCmds.accel_cmd = 0;
    ActCmds.decel_cmd = ActReq.a_des;
end

psi_des = unwrap(psi_des);
Ctl.IdealSensors.psi = unwrap(Ctl.IdealSensors.psi);

ActCmds.steering_cmd = 3.5*(psi_des - Ctl.IdealSensors.psi);

== matlab function SingleVehicle_01/VehicleDynamics/KinematicVehicleModel ==
  data: u input double; delta input double; dX output double; psi input double; dY output double; dpsi output double; veh_struct parameter double
function [dX,dY,dpsi] = fcn(u,delta, psi, veh_struct)

lf = veh_struct.lf;
lr = veh_struct.lr;

% psi = unwrap(psi);
% delta = unwrap(delta);

beta = atan( lr /(lf + lr) * tan(delta));

% beta = unwrap(beta);

dX = u * cos(psi + beta);
dY = u * sin(psi + beta);
dpsi = u / lr * sin(beta);

== matlab function SingleVehicle_01/Controller/Actuation/ActuatorDrivers ==
  data: ActCmds input Bus: ActuationCmdBus; accel_cmd output double; decel_cmd output double; steering_cmd output double
function [accel_cmd, decel_cmd, steering_cmd]  = fcn(ActCmds)

accel_cmd = ActCmds.accel_cmd;
decel_cmd = ActCmds.decel_cmd;
steering_cmd = ActCmds.steering_cmd;

end

== matlab function SingleVehicle_01/Controller/FeaturedFunctions/wPFollower/calcDesdCmds ==
  data: prevWpAction input Bus: wpFollower; prevSituation input Bus: situationBus; wpAction output Bus: wpFollower; veh_struct parameter double; newSituation output Bus: situationBus
function [wpAction, newSituation] = wpFollower(prevWpAction, prevSituation, veh_struct)


%waypoint Definition
currentIndex = prevSituation.wP.currentWayPointIndex;
if currentIndex < 1
    currentIndex = uint16(1);
end
finalIndex = prevSituation.wP.finalWayPointIndex;

xd = prevSituation.wP.wayPointArray(currentIndex).x;
yd = prevSituation.wP.wayPointArray(currentIndex).y;
xa = prevSituation.selfAwarenessBus.x;
ya = prevSituation.selfAwarenessBus.y;
howClose = norm([xd-xa, yd-ya]);

if howClose < veh_struct.wpControl.wayPointThreshold
    if (currentIndex == finalIndex)
        currentIndex = uint16(1);
    else
        currentIndex = uint16(currentIndex + 1);
    end
end

newSituation = prevSituation;
newSituation.wP.currentWayPointIndex = uint16(currentIndex);
newSituation.wP.currentWayPoint.x = newSituation.wP.wayPointArray(currentIndex).x;
newSituation.wP.currentWayPoint.y = newSituation.wP.wayPointArray(currentIndex).y;
newSituation.wP.currentWayPoint.z = newSituation.wP.wayPointArray(currentIndex).z;
newSituation.wP.currentWayPoint.treach = newSituation.wP.wayPointArray(currentIndex).treach;


%New Way POint Definition

newSituation = prevSituation;
newSituation.wP.currentWayPointIndex = uint16(currentIndex);
newSituation.wP.currentWayPoint.x = ControllerBus.ConnectedBus.ObjectBus.x;
newSituation.wP.currentWayPoint.y = ControllerBus.ConnectedBus.ObjectBus.y;
newSituation.wP.currentWayPoint.z = ControllerBus.ConnectedBus.ObjectBus.z;
newSituation.wP.currentWayPoint.treach = 0;


%wayPoint Following Algorithm

v_des_raw = min(veh_struct.wpControl.v_des_max, howClose / veh_struct.wpControl.howClose_saturate * veh_struct.wpControl.v_des_max);
psi_des_raw = atan2((yd-ya),(xd-xa));

% if psi_des_raw < 0
%     
%     dbg = 1;
%     
% end
    

v_des_old = prevWpAction.v_des;
psi_des_old = prevWpAction.psi_des;

a_des = veh_struct.wpControl.v_des_filter.lambda * (v_des_raw - v_des_old);
v_des = v_des_old + veh_struct.CONTROL_OS_SAMPLETIME * a_des;

dpsi_des = veh_struct.wpControl.psi_des_filter.lambda * (psi_des_raw - psi_des_old);
psi_des = psi_des_old + veh_struct.CONTROL_OS_SAMPLETIME * dpsi_des;
% psi_des = mod(psi_des, 2 * pi);


wpAction.v_des = v_des;
wpAction.a_des = a_des;
wpAction.psi_des = psi_des;
wpAction.dpsi_des = dpsi_des;

end

== matlab function SingleVehicle_01/Controller/FeaturedFunctions/wPFollower/defineWayPointsNewWay ==
  data: prevWpAction input Bus: wpFollower; prevSituation input Bus: situationBus; wpAction output Bus: wpFollower; veh_struct parameter double; newSituation output Bus: situationBus
function [wpAction, newSituation] = wpFollower(prevWpAction, prevSituation, veh_struct)


%waypoint Definition
currentIndex = prevSituation.wP.currentWayPointIndex;
if currentIndex < 1
    currentIndex = uint16(1);
end
finalIndex = prevSituation.wP.finalWayPointIndex;

xd = prevSituation.wP.wayPointArray(currentIndex).x;
yd = prevSituation.wP.wayPointArray(currentIndex).y;
xa = prevSituation.selfAwarenessBus.x;
ya = prevSituation.selfAwarenessBus.y;
howClose = norm([xd-xa, yd-ya]);

if howClose < veh_struct.wpControl.wayPointThreshold
    if (currentIndex == finalIndex)
        currentIndex = uint16(1);
    else
        currentIndex = uint16(currentIndex + 1);
    end
end

newSituation = prevSituation;
newSituation.wP.currentWayPointIndex = uint16(currentIndex);
newSituation.wP.currentWayPoint.x = newSituation.wP.wayPointArray(currentIndex).x;
newSituation.wP.currentWayPoint.y = newSituation.wP.wayPointArray(currentIndex).y;
newSituation.wP.currentWayPoint.z = newSituation.wP.wayPointArray(currentIndex).z;
newSituation.wP.currentWayPoint.treach = newSituation.wP.wayPointArray(currentIndex).treach;


%New Way POint Definition

newSituation = prevSituation;
newSituation.wP.currentWayPointIndex = uint16(currentIndex);
newSituation.wP.currentWayPoint.x = ControllerBus.ConnectedBus.ObjectBus.x;
newSituation.wP.currentWayPoint.y = ControllerBus.ConnectedBus.ObjectBus.y;
newSituation.wP.currentWayPoint.z = ControllerBus.ConnectedBus.ObjectBus.z;
newSituation.wP.currentWayPoint.treach = 0;


%wayPoint Following Algorithm

v_des_raw = min(veh_struct.wpControl.v_des_max, howClose / veh_struct.wpControl.howClose_saturate * veh_struct.wpControl.v_des_max);
psi_des_raw = atan2((yd-ya),(xd-xa));

% if psi_des_raw < 0
%     
%     dbg = 1;
%     
% end
    

v_des_old = prevWpAction.v_des;
psi_des_old = prevWpAction.psi_des;

a_des = veh_struct.wpControl.v_des_filter.lambda * (v_des_raw - v_des_old);
v_des = v_des_old + veh_struct.CONTROL_OS_SAMPLETIME * a_des;

dpsi_des = veh_struct.wpControl.psi_des_filter.lambda * (psi_des_raw - psi_des_old);
psi_des = psi_des_old + veh_struct.CONTROL_OS_SAMPLETIME * dpsi_des;
% psi_des = mod(psi_des, 2 * pi);


wpAction.v_des = v_des;
wpAction.a_des = a_des;
wpAction.psi_des = psi_des;
wpAction.dpsi_des = dpsi_des;

end
